simulink library "GPS_INS_Block"  (R2018b)
settings: Solver=VariableStepAuto  StartTime=0.0  StopTime=10.0  RelTol=1e-3
undefined symbols (not defined in the file): ac1dyn_alt0_ft, ac1dyn_lat0_rad, ac1dyn_lon0_rad, magnitude, uas_own_altQuant_ft, uas_own_dt_s, uas_own_phi_random_stddev_rad, uas_own_psi_random_stddev_rad, uas_own_seed1, uas_own_seed10, uas_own_seed2, uas_own_seed3, uas_own_seed4, uas_own_seed5, uas_own_seed6, uas_own_seed7, uas_own_seed8, uas_own_seed9, uas_own_theta_random_stddev_rad, uas_own_usePerfectAlt, uas_own_vx_bias_ftps, uas_own_vx_random_stddev_ftps, uas_own_vx_tau_s, uas_own_vy_bias_ftps, uas_own_vy_random_stddev_ftps, uas_own_vy_tau_s, uas_own_x_bias_ft, uas_own_x_random_stddev_ft, uas_own_x_tau_s, uas_own_y_bias_ft, uas_own_y_random_stddev_ft, uas_own_y_tau_s
libraries: simulink x4, TSAA_AltRate_Error x1, TSAA_Altitude_Error x1
settings Model: Creator=RA24876  LastModifiedBy=BI28030
settings SFSimCC: SimUseLocalCustomCode=off
settings RTWCC: RTWUseLocalCustomCode=off
settings CodeAppCC: StateflowObjectComments=on

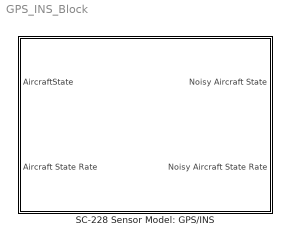
== system GPS_INS_Block ==
  SC-228 Sensor Model: GPS/INS : Subsystem  mask(Own State: GPS){dt_s=uas_own_dt_s, perfect=uas_own_usePerfectAlt, lat0_rad=ac1dyn_lat0_rad, lon0_rad=ac1dyn_lon0_rad, alt0_ft=ac1dyn_alt0_ft, vx_random_stddev_ftps=uas_own_vy_random_stddev_ftps, vx_bias_ftps=uas_own_vy_bias_ftps, vx_tau_s=uas_own_vy_tau_s, seed4=uas_own_seed4, vy_random_stddev_ftps=uas_own_vx_random_stddev_ftps, vy_bias_ftps=uas_own_vx_bias_ftps, vy_tau_s=uas_own_vx_tau_s, seed5=uas_own_seed5, psi_random_stddev_rad=uas_own_psi_random_stddev_rad, seed1=uas_own_seed1, phi_random_stddev_rad=uas_own_phi_random_stddev_rad, seed2=uas_own_seed2, theta_random_stddev_rad=uas_own_theta_random_stddev_rad, seed3=uas_own_seed3, seed6=uas_own_seed6, y_random_stddev_ft=uas_own_y_random_stddev_ft, y_bias_ft=uas_own_y_bias_ft, y_tau_s=uas_own_y_tau_s, seed7=uas_own_seed7, x_random_stddev_ft=uas_own_x_random_stddev_ft, x_bias_ft=uas_own_x_bias_ft, x_tau_s=uas_own_x_tau_s, seed8=uas_own_seed8, seed9=uas_own_seed9, seed10=uas_own_seed10, altQuant_ft=uas_own_altQuant_ft}
      mask prompts: dt_s "Timestep (s)"; perfect "Use Perfect Altimetry?"; lat0_rad "ENU Reference Latitude (rad)"; lon0_rad "ENU Reference Longitude (rad)"; alt0_ft "ENU Reference Altitude (ft)"; vx_random_stddev_ftps "Random Error Standard Deviation (ft/s)"; vx_bias_ftps "Bias Error (ft/s)"; vx_tau_s "Correlation Time (s)"; seed4 "Random Seed"; vy_random_stddev_ftps "Random Error Standard Deviation (ft/s)"; vy_bias_ftps "Bias Error (ft/s)"; vy_tau_s "Correlation Time (s)"; seed5 "Random Seed"; psi_random_stddev_rad "Random Error Standard Deviation (rad)"; seed1 "Random Seed"; phi_random_stddev_rad "Random Error Standard Deviation (rad)"; seed2 "Random Seed"; theta_random_stddev_rad "Random Error Standard Deviation (rad)"; seed3 "Random Seed"; seed6 "Random Seed"; y_random_stddev_ft "Random Error Standard Deviation (ft)"; y_bias_ft "Bias Error (ft)"; y_tau_s "Correlation Time (s)"; seed7 "Random Seed"; x_random_stddev_ft "Random Error Standard Deviation (ft)"; x_bias_ft "Bias Error (ft)"; x_tau_s "Correlation Time (s)"; seed8 "Random Seed"; seed9 "Lambda Random Seed"; seed10 "Random Seed"; altQuant_ft "Altitude Quantization"
      mask help: Ownship navigation error model with colored noise with state and state rate output.
      mask Help:
      | Additive noise model of ownship GPS navigation.  Independent noise is added to
      | each of latitude, longitude, and altitude and their rates as well as vertical acceleration,
      | heading, roll, and roll rate parameters. Noise is colored using weights determined
      | by time constant parameters.
      | 
      | Output takes the form of AircraftState and AircraftStateRate data buses.
      mask DialogControl ParameterTabVar0 Prompt: Tab
      mask DialogControl ParameterTabVar01234 Prompt: Velocity (N)
      mask DialogControl ParameterTabVar012345 Prompt: Velocity (E)
      mask DialogControl ParameterTabVar012345678 Prompt: Heading
      mask DialogControl ParameterTabVar0123456789 Prompt: Roll
      mask DialogControl ParameterTabVar012345678910 Prompt: Pitch
      mask DialogControl ParameterTabVar012345678911 Prompt: Vertical Rate
      mask DialogControl ParameterTabVar012345678912 Prompt: Position (N)
      mask DialogControl ParameterTabVar012345678913 Prompt: Position (E)
      mask DialogControl ParameterTabVar012345678914 Prompt: Position (h)

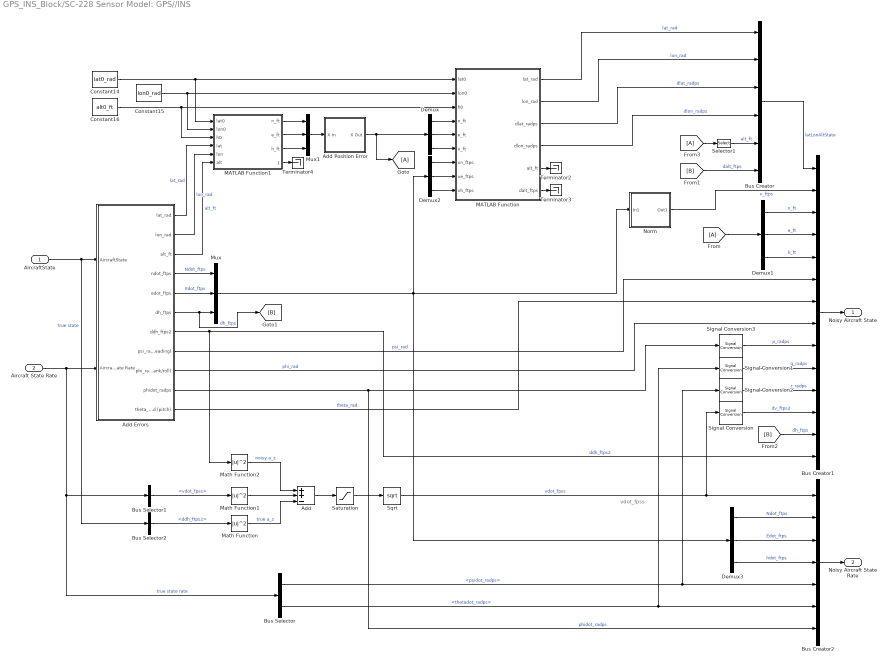
== system GPS_INS_Block/SC-228 Sensor Model: GPS//INS ==
  note: vdot_fpss
  AircraftState : Inport  OutDataTypeStr=Bus: AircraftState
  Aircraft State Rate : Inport  Port=2  OutDataTypeStr=Bus: AircraftStateRate
  Add : Sum  Inputs=++-
  Add Errors : Subsystem
  Add Position Error : Subsystem
  Bus Creator : BusCreator  Inputs=6  OutDataTypeStr=Bus: LatLonAltMeasurement
  Bus Creator1 : BusCreator  Inputs=14  OutDataTypeStr=Bus: AircraftState
  Bus Creator2 : BusCreator  Inputs=7  OutDataTypeStr=Bus: AircraftStateRate
  Bus Selector : BusSelector  OutputSignals=psidot_radps,thetadot_radps
  Bus Selector1 : BusSelector  OutputSignals=vdot_fpss
  Bus Selector2 : BusSelector  OutputSignals=ddh_ftps2
  Constant14 : Constant  Value=lat0_rad  OutDataTypeStr=double
  Constant15 : Constant  Value=lon0_rad  OutDataTypeStr=double
  Constant16 : Constant  Value=alt0_ft  OutDataTypeStr=double
  Demux{,1..3} (4 alike) : Demux  Outputs=3
  MATLAB Function : MATLAB Function  TreatAsAtomicUnit=on
  MATLAB Function1 : MATLAB Function  TreatAsAtomicUnit=on
  Math Function : Math  Operator=magnitude^2  SaturateOnIntegerOverflow=on
  Math Function1 : Math  Operator=magnitude^2  SaturateOnIntegerOverflow=on
  Math Function2 : Math  Operator=magnitude^2  SaturateOnIntegerOverflow=on
  Mux : Mux  Inputs=3
  Mux1 : Mux  Inputs=3
  Norm : Subsystem
  Saturation : Saturate  UpperLimit=Inf  LowerLimit=0
  Selector1 : Selector  InputPortWidth=3  IndexOptions=Index vector (dialog)  Indices=[3]  OutputSizes=1
  Signal Conversion{,1..3} (4 alike) : SignalConversion  OverrideOpt=off
  Sqrt : Sqrt  SaturateOnIntegerOverflow=on
  Terminator2 : Terminator
  Terminator3 : Terminator
  Terminator4 : Terminator
  Noisy Aircraft State : Outport  OutDataTypeStr=Bus: AircraftState
  Noisy Aircraft State Rate : Outport  Port=2  OutDataTypeStr=Bus: AircraftStateRate
  wires:
  Signal Conversion3/1 -> Bus Creator1/9  "p_radps"
  Signal Conversion2/1 -> Bus Creator1/11  "r_radps"
  Signal Conversion1/1 -> Bus Creator1/10  "q_radps"
  Add Errors/11(theta_rad (pitch)) -> Bus Creator1/7  "theta_rad"
  [B] -> Bus Creator1/13  "dh_ftps"
  [B] -> Bus Creator/6  "dalt_ftps"
  Demux3/3 -> Bus Creator2/4  "hdot_ftps"
  Demux3/2 -> Bus Creator2/3  "Edot_ftps"
  Demux3/1 -> Bus Creator2/2  "Ndot_ftps"
  Demux2/3 -> MATLAB Function/9(vh_ftps)
  Demux2/2 -> MATLAB Function/8(ve_ftps)
  Demux2/1 -> MATLAB Function/7(vn_ftps)
  Demux1/1 -> Bus Creator1/3  "n_ft"
  Demux1/2 -> Bus Creator1/4  "e_ft"
  Demux1/3 -> Bus Creator1/5  "h_ft"
  Mux1/1 -> Add Position Error/1(X In)
  Demux/3 -> MATLAB Function/6(u_ft)
  Demux/2 -> MATLAB Function/5(e_ft)
  Demux/1 -> MATLAB Function/4(n_ft)
  Signal Conversion/1 -> Bus Creator1/12  "dv_ftps2"
  Norm/1(Out1) -> Bus Creator1/2  "v_ftps"
  Mux/1 -> Demux3/1, Norm/1(In1), Demux2/1
  Sqrt/1 -> Signal Conversion/1, Bus Creator2/1  "vdot_fpss"
  Add/1 -> Saturation/1
  Math Function/1 -> Add/3  "true a_z"
  Math Function2/1 -> Add/1  "noisy a_z"
  Math Function1/1 -> Add/2
  Bus Selector2/1 -> Math Function/1  "<ddh_ftps2>"
  Bus Selector1/1 -> Math Function1/1  "<vdot_fpss>"
  Constant14/1 -> MATLAB Function1/1(lat0), MATLAB Function/1(lat0)
  Constant15/1 -> MATLAB Function1/2(lon0), MATLAB Function/2(lon0)
  Constant16/1 -> MATLAB Function1/3(h0), MATLAB Function/3(h0)
  MATLAB Function1/3(h_ft) -> Mux1/3
  MATLAB Function1/2(e_ft) -> Mux1/2
  MATLAB Function1/1(n_ft) -> Mux1/1
  MATLAB Function1/4(J) -> Terminator4/1
  MATLAB Function/4(dlon_radps) -> Bus Creator/4  "dlon_radps"
  MATLAB Function/3(dlat_radps) -> Bus Creator/3  "dlat_radps"
  Bus Selector/2 -> Bus Creator2/6, Signal Conversion1/1  "<thetadot_radps>"
  Bus Selector/1 -> Signal Conversion2/1, Bus Creator2/5  "<psidot_radps>"
  Add Errors/5(edot_ftps) -> Mux/2  "Edot_ftps"
  Add Errors/4(ndot_ftps) -> Mux/1  "Ndot_ftps"
  Bus Creator2/1 -> Noisy Aircraft State Rate/1
  Bus Creator1/1 -> Noisy Aircraft State/1
  Bus Creator/1 -> Bus Creator1/1  "latLonAltState"
  MATLAB Function/6(dalt_ftps) -> Terminator3/1
  MATLAB Function/5(alt_ft) -> Terminator2/1
  Add Errors/6(dh_ftps) -> Mux/3, [B]  "dh_ftps"
  Add Errors/3(alt_ft) -> MATLAB Function1/6(alt)  "alt_ft"
  Add Errors/2(lon_rad) -> MATLAB Function1/5(lon)  "lon_rad"
  Add Errors/1(lat_rad) -> MATLAB Function1/4(lat)  "lat_rad"
  Add Errors/10(phidot_radps) -> Bus Creator2/7, Signal Conversion3/1  "phidot_radps"
  Add Errors/9(phi_rad (bank/roll)) -> Bus Creator1/8  "phi_rad"
  Add Errors/8(psi_rad (heading)) -> Bus Creator1/6  "psi_rad"
  Add Errors/7(ddh_ftps2) -> Bus Creator1/14, Math Function2/1  "ddh_ftps2"
  Aircraft State Rate/1 -> Add Errors/2(Aircraft State Rate), Bus Selector1/1, Bus Selector/1  "true state rate"
  AircraftState/1 -> Add Errors/1(AircraftState), Bus Selector2/1  "true state"
  Saturation/1 -> Sqrt/1
  Add Position Error/1(X Out) -> Demux/1, [A]
  [A] -> Selector1/1
  Selector1/1 -> Bus Creator/5  "alt_ft"
  [A] -> Demux1/1
  MATLAB Function/1(lat_rad) -> Bus Creator/1  "lat_rad"
  MATLAB Function/2(lon_rad) -> Bus Creator/2  "lon_rad"

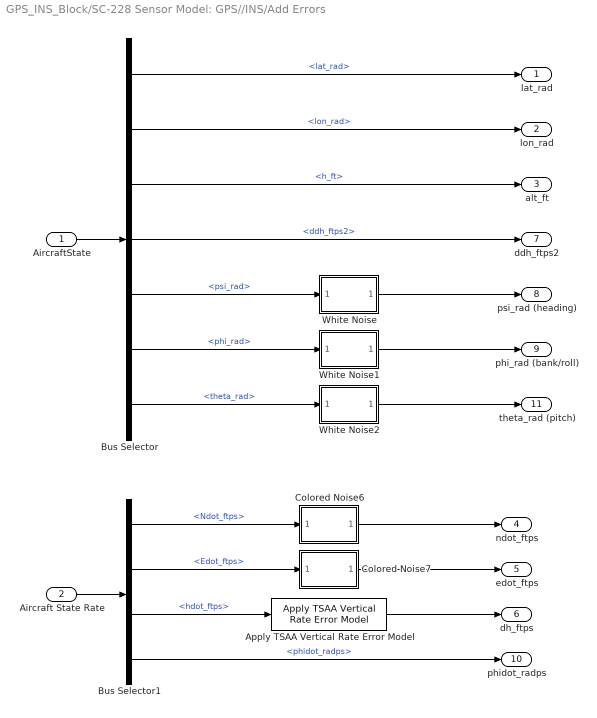
== system GPS_INS_Block/SC-228 Sensor Model: GPS//INS/Add Errors ==
  AircraftState : Inport  OutDataTypeStr=Bus: AircraftState
  Aircraft State Rate : Inport  Port=2  OutDataTypeStr=Bus: AircraftStateRate
  Apply TSAA Vertical Rate Error Model : TSAA_AltRate_Error/Apply TSAA Vertical Rate Error Model  perfect=perfect  seed=seed6  dt_s=dt_s
  Bus Selector : BusSelector  OutputSignals=latLonAltState.lat_rad,latLonAltState.lon_rad,h_ft,ddh_ftps2,psi_rad,phi_rad,theta_rad
  Bus Selector1 : BusSelector  OutputSignals=Ndot_ftps,Edot_ftps,hdot_ftps,phidot_radps
  Colored Noise6 : Subsystem  mask(Colored Noise){sig=vy_random_stddev_ftps, bias=vy_bias_ftps, tau=vy_tau_s, dt=dt_s, seed=seed4}
      mask prompts: sig "Random error standard deviation"; bias "Bias error"; tau "Correlation time"; dt "Track update time"; seed "Random Seed"
      mask help: Generates a noisy state variable estimate using the ABSAA colored noise model. Set correlation time to zero for white noise.
      mask Help:
      | Generates a noisy state variable estimate using the AF Common ABSAA error
      | model.  Time correlation of the error is defined by an exponential decay
      | of K = exp(-tau/dt), where tau is the correlation time and dt is the time
      | between track updates.  The track error at time t is then:
      | 
      |     err(t) = K*err(t-1) + N(0,(1-K^2)*sig^2) + bias
      | 
      | where N(x,y) is a Gaussian noise process with mean x and variance y and
      | with random number generator seeded with the integer 'seed'.
      | 
      | The random noise process must be initialized with an error drawn from
      | N(0,sig^2).
      | 
      | The noise model can be used to produce white noise by setting tau to zero.
  Colored Noise7 : Subsystem  mask(Colored Noise){sig=vx_random_stddev_ftps, bias=vx_bias_ftps, tau=vx_tau_s, dt=dt_s, seed=seed5}
      mask prompts: sig "Random error standard deviation"; bias "Bias error"; tau "Correlation time"; dt "Track update time"; seed "Random Seed"
      mask help: Generates a noisy state variable estimate using the ABSAA colored noise model. Set correlation time to zero for white noise.
      mask Help:
      | Generates a noisy state variable estimate using the AF Common ABSAA error
      | model.  Time correlation of the error is defined by an exponential decay
      | of K = exp(-tau/dt), where tau is the correlation time and dt is the time
      | between track updates.  The track error at time t is then:
      | 
      |     err(t) = K*err(t-1) + N(0,(1-K^2)*sig^2) + bias
      | 
      | where N(x,y) is a Gaussian noise process with mean x and variance y and
      | with random number generator seeded with the integer 'seed'.
      | 
      | The random noise process must be initialized with an error drawn from
      | N(0,sig^2).
      | 
      | The noise model can be used to produce white noise by setting tau to zero.
  White Noise : Subsystem  mask(Colored Noise){sig=psi_random_stddev_rad, seed=seed1}
      mask prompts: sig "Random error standard deviation"; seed "Random Seed"
      mask help: Generates a noisy state variable estimate using the ABSAA colored noise model. Set correlation time to zero for white noise.
      mask Help:
      | Generates a noisy state variable estimate using the AF Common ABSAA error
      | model.  Time correlation of the error is defined by an exponential decay
      | of K = exp(-tau/dt), where tau is the correlation time and dt is the time
      | between track updates.  The track error at time t is then:
      | 
      |     err(t) = K*err(t-1) + N(0,(1-K^2)*sig^2) + bias
      | 
      | where N(x,y) is a Gaussian noise process with mean x and variance y and
      | with random number generator seeded with the integer 'seed'.
      | 
      | The random noise process must be initialized with an error drawn from
      | N(0,sig^2).
      | 
      | The noise model can be used to produce white noise by setting tau to zero.
  White Noise1 : Subsystem  mask(Colored Noise){sig=phi_random_stddev_rad, seed=seed2}
      mask prompts: sig "Random error standard deviation"; seed "Random Seed"
      mask help: Generates a noisy state variable estimate using the ABSAA colored noise model. Set correlation time to zero for white noise.
      mask Help:
      | Generates a noisy state variable estimate using the AF Common ABSAA error
      | model.  Time correlation of the error is defined by an exponential decay
      | of K = exp(-tau/dt), where tau is the correlation time and dt is the time
      | between track updates.  The track error at time t is then:
      | 
      |     err(t) = K*err(t-1) + N(0,(1-K^2)*sig^2) + bias
      | 
      | where N(x,y) is a Gaussian noise process with mean x and variance y and
      | with random number generator seeded with the integer 'seed'.
      | 
      | The random noise process must be initialized with an error drawn from
      | N(0,sig^2).
      | 
      | The noise model can be used to produce white noise by setting tau to zero.
  White Noise2 : Subsystem  mask(Colored Noise){sig=theta_random_stddev_rad, seed=seed3}
      mask prompts: sig "Random error standard deviation"; seed "Random Seed"
      mask help: Generates a noisy state variable estimate using the ABSAA colored noise model. Set correlation time to zero for white noise.
      mask Help:
      | Generates a noisy state variable estimate using the AF Common ABSAA error
      | model.  Time correlation of the error is defined by an exponential decay
      | of K = exp(-tau/dt), where tau is the correlation time and dt is the time
      | between track updates.  The track error at time t is then:
      | 
      |     err(t) = K*err(t-1) + N(0,(1-K^2)*sig^2) + bias
      | 
      | where N(x,y) is a Gaussian noise process with mean x and variance y and
      | with random number generator seeded with the integer 'seed'.
      | 
      | The random noise process must be initialized with an error drawn from
      | N(0,sig^2).
      | 
      | The noise model can be used to produce white noise by setting tau to zero.
  lat_rad : Outport
  lon_rad : Outport  Port=2
  alt_ft : Outport  Port=3
  ndot_ftps : Outport  Port=4
  edot_ftps : Outport  Port=5
  dh_ftps : Outport  Port=6
  ddh_ftps2 : Outport  Port=7
  psi_rad (heading) : Outport  Port=8
  phi_rad (bank/roll) : Outport  Port=9
  phidot_radps : Outport  Port=10
  theta_rad (pitch) : Outport  Port=11
  wires:
  Bus Selector1/1 -> Colored Noise6/1(truth)  "<Ndot_ftps>"
  Bus Selector1/2 -> Colored Noise7/1(truth)  "<Edot_ftps>"
  Bus Selector1/3 -> Apply TSAA Vertical Rate Error Model/1  "<hdot_ftps>"
  Bus Selector1/4 -> phidot_radps/1  "<phidot_radps>"
  Aircraft State Rate/1 -> Bus Selector1/1
  Colored Noise6/1(noisy) -> ndot_ftps/1
  White Noise/1(noisy) -> psi_rad (heading)/1
  Bus Selector/4 -> ddh_ftps2/1  "<ddh_ftps2>"
  Bus Selector/1 -> lat_rad/1  "<lat_rad>"
  Colored Noise7/1(noisy) -> edot_ftps/1
  AircraftState/1 -> Bus Selector/1
  Bus Selector/6 -> White Noise1/1(truth)  "<phi_rad>"
  Bus Selector/2 -> lon_rad/1  "<lon_rad>"
  Bus Selector/5 -> White Noise/1(truth)  "<psi_rad>"
  White Noise1/1(noisy) -> phi_rad (bank/roll)/1
  Bus Selector/3 -> alt_ft/1  "<h_ft>"
  Apply TSAA Vertical Rate Error Model/1 -> dh_ftps/1
  Bus Selector/7 -> White Noise2/1(truth)  "<theta_rad>"
  White Noise2/1(noisy) -> theta_rad (pitch)/1

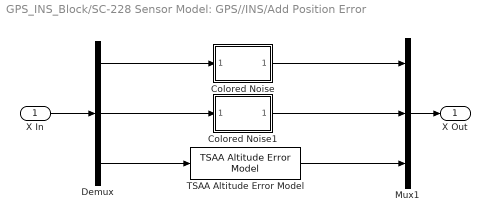
== system GPS_INS_Block/SC-228 Sensor Model: GPS//INS/Add Position Error ==
  X In : Inport
  Colored Noise : Subsystem  mask(Colored Noise){sig=y_random_stddev_ft, bias=y_bias_ft, tau=y_tau_s, dt=dt_s, seed=seed7}
      mask prompts: sig "Random error standard deviation"; bias "Bias error"; tau "Correlation time"; dt "Track update time"; seed "Random Seed"
      mask help: Generates a noisy state variable estimate using the ABSAA colored noise model. Set correlation time to zero for white noise.
      mask Help:
      | Generates a noisy state variable estimate using the AF Common ABSAA error
      | model.  Time correlation of the error is defined by an exponential decay
      | of K = exp(-tau/dt), where tau is the correlation time and dt is the time
      | between track updates.  The track error at time t is then:
      | 
      |     err(t) = K*err(t-1) + N(0,(1-K^2)*sig^2) + bias
      | 
      | where N(x,y) is a Gaussian noise process with mean x and variance y and
      | with random number generator seeded with the integer 'seed'.
      | 
      | The random noise process must be initialized with an error drawn from
      | N(0,sig^2).
      | 
      | The noise model can be used to produce white noise by setting tau to zero.
  Colored Noise1 : Subsystem  mask(Colored Noise){sig=x_random_stddev_ft, bias=x_bias_ft, tau=x_tau_s, dt=dt_s, seed=seed8}
      mask prompts: sig "Random error standard deviation"; bias "Bias error"; tau "Correlation time"; dt "Track update time"; seed "Random Seed"
      mask help: Generates a noisy state variable estimate using the ABSAA colored noise model. Set correlation time to zero for white noise.
      mask Help:
      | Generates a noisy state variable estimate using the AF Common ABSAA error
      | model.  Time correlation of the error is defined by an exponential decay
      | of K = exp(-tau/dt), where tau is the correlation time and dt is the time
      | between track updates.  The track error at time t is then:
      | 
      |     err(t) = K*err(t-1) + N(0,(1-K^2)*sig^2) + bias
      | 
      | where N(x,y) is a Gaussian noise process with mean x and variance y and
      | with random number generator seeded with the integer 'seed'.
      | 
      | The random noise process must be initialized with an error drawn from
      | N(0,sig^2).
      | 
      | The noise model can be used to produce white noise by setting tau to zero.
  Demux : Demux  Outputs=3
  Mux1 : Mux  Inputs=3
  TSAA Altitude Error Model : TSAA_Altitude_Error/TSAA Altitude Error Model  ac_id=1  perfect=perfect  lambdaSeed=seed9  randomSeed=seed10  altQuant_ft=altQuant_ft  dt_s=dt_s
  X Out : Outport
  wires:
  Mux1/1 -> X Out/1
  X In/1 -> Demux/1
  Demux/3 -> TSAA Altitude Error Model/1
  TSAA Altitude Error Model/1 -> Mux1/3
  Demux/1 -> Colored Noise/1(truth)
  Colored Noise/1(noisy) -> Mux1/1
  Demux/2 -> Colored Noise1/1(truth)
  Colored Noise1/1(noisy) -> Mux1/2

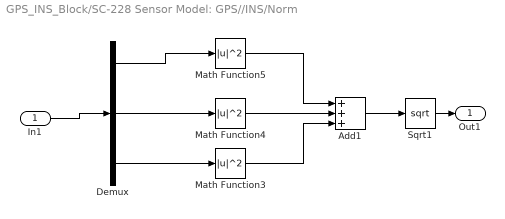
== system GPS_INS_Block/SC-228 Sensor Model: GPS//INS/Norm ==
  In1 : Inport
  Add1 : Sum  Inputs=+++
  Demux : Demux  Outputs=3
  Math Function3 : Math  Operator=magnitude^2  SaturateOnIntegerOverflow=on
  Math Function4 : Math  Operator=magnitude^2  SaturateOnIntegerOverflow=on
  Math Function5 : Math  Operator=magnitude^2  SaturateOnIntegerOverflow=on
  Sqrt1 : Sqrt  SaturateOnIntegerOverflow=on
  Out1 : Outport
  wires:
  In1/1 -> Demux/1
  Demux/2 -> Math Function4/1
  Math Function3/1 -> Add1/3
  Math Function4/1 -> Add1/2
  Math Function5/1 -> Add1/1
  Demux/3 -> Math Function3/1
  Sqrt1/1 -> Out1/1
  Demux/1 -> Math Function5/1
  Add1/1 -> Sqrt1/1

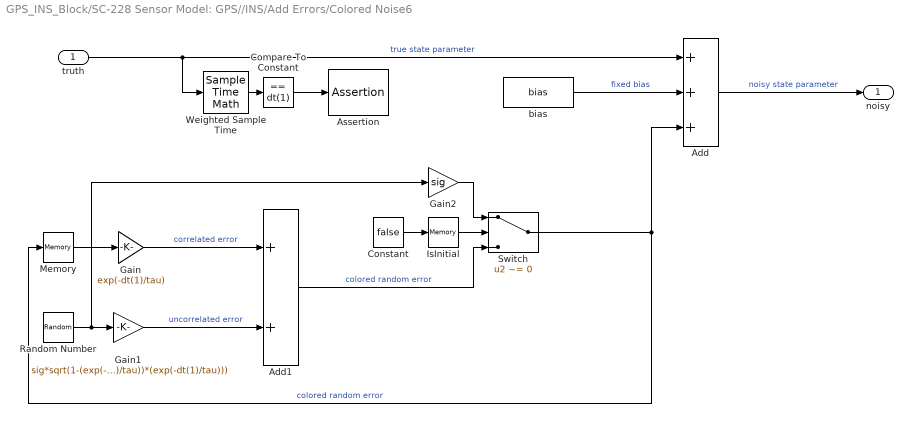
== system GPS_INS_Block/SC-228 Sensor Model: GPS//INS/Add Errors/Colored Noise6 ==
  truth : Inport
  Add : Sum  Inputs=+++  SampleTime=dt_s
  Add1 : Sum  SampleTime=dt
  Assertion : Assertion
  Compare To Constant : simulink/Logic and Bit Operations/Compare To Constant  relop===  const=dt(1)  OutDataTypeStr=boolean
  Constant : Constant  Value=false
  Gain : Gain  Gain=exp(-dt(1)/tau)  SampleTime=dt
  Gain1 : Gain  Gain=sig*sqrt(1-(exp(-dt(1)/tau))*(exp(-dt(1)/tau)))
  Gain2 : Gain  Gain=sig
  IsInitial : Memory  InitialCondition=true  InheritSampleTime=on
  Memory : Memory  InheritSampleTime=on
  Random Number : RandomNumber  Seed=seed  SampleTime=dt_s
  Switch : Switch  Criteria=u2 ~= 0  SampleTime=dt
  Weighted Sample Time : SampleTimeMath  TsampMathOp=Ts Only
  bias : Constant  Value=bias
  noisy : Outport
  wires:
  Compare To Constant/1 -> Assertion/1
  Weighted Sample Time/1 -> Compare To Constant/1
  Gain2/1 -> Switch/1
  Add1/1 -> Switch/3  "colored random error"
  IsInitial/1 -> Switch/2
  Constant/1 -> IsInitial/1
  Memory/1 -> Gain/1
  truth/1 -> Add/1, Weighted Sample Time/1  "true state parameter"
  Add/1 -> noisy/1  "noisy state parameter"
  Gain/1 -> Add1/1  "correlated error"
  Random Number/1 -> Gain1/1, Gain2/1
  bias/1 -> Add/2  "fixed bias"
  Switch/1 -> Add/3, Memory/1  "colored random error"
  Gain1/1 -> Add1/2  "uncorrelated error"

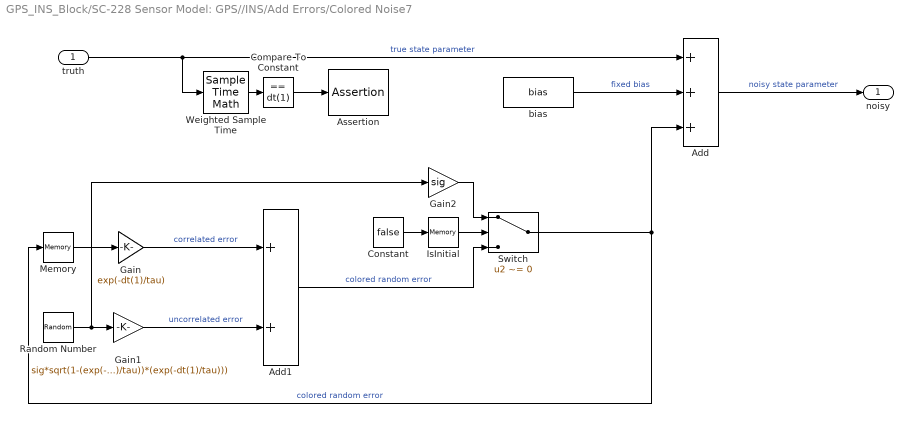
== system GPS_INS_Block/SC-228 Sensor Model: GPS//INS/Add Errors/Colored Noise7 ==
  truth : Inport
  Add : Sum  Inputs=+++  SampleTime=dt_s
  Add1 : Sum  SampleTime=dt
  Assertion : Assertion
  Compare To Constant : simulink/Logic and Bit Operations/Compare To Constant  relop===  const=dt(1)  OutDataTypeStr=boolean
  Constant : Constant  Value=false
  Gain : Gain  Gain=exp(-dt(1)/tau)  SampleTime=dt
  Gain1 : Gain  Gain=sig*sqrt(1-(exp(-dt(1)/tau))*(exp(-dt(1)/tau)))
  Gain2 : Gain  Gain=sig
  IsInitial : Memory  InitialCondition=true  InheritSampleTime=on
  Memory : Memory  InheritSampleTime=on
  Random Number : RandomNumber  Seed=seed  SampleTime=dt_s
  Switch : Switch  Criteria=u2 ~= 0  SampleTime=dt
  Weighted Sample Time : SampleTimeMath  TsampMathOp=Ts Only
  bias : Constant  Value=bias
  noisy : Outport
  wires:
  Compare To Constant/1 -> Assertion/1
  Weighted Sample Time/1 -> Compare To Constant/1
  Gain2/1 -> Switch/1
  Add1/1 -> Switch/3  "colored random error"
  IsInitial/1 -> Switch/2
  Constant/1 -> IsInitial/1
  Memory/1 -> Gain/1
  truth/1 -> Add/1, Weighted Sample Time/1  "true state parameter"
  Add/1 -> noisy/1  "noisy state parameter"
  Gain/1 -> Add1/1  "correlated error"
  Random Number/1 -> Gain1/1, Gain2/1
  bias/1 -> Add/2  "fixed bias"
  Switch/1 -> Add/3, Memory/1  "colored random error"
  Gain1/1 -> Add1/2  "uncorrelated error"

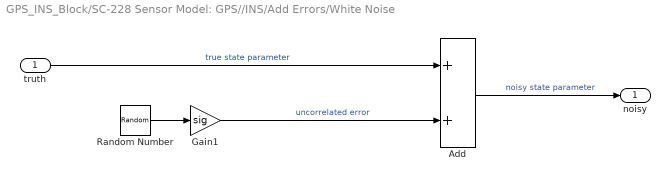
== system GPS_INS_Block/SC-228 Sensor Model: GPS//INS/Add Errors/White Noise ==
  truth : Inport
  Add : Sum  SampleTime=dt_s
  Gain1 : Gain  Gain=sig
  Random Number : RandomNumber  Seed=seed  SampleTime=dt_s
  noisy : Outport
  wires:
  truth/1 -> Add/1  "true state parameter"
  Add/1 -> noisy/1  "noisy state parameter"
  Random Number/1 -> Gain1/1
  Gain1/1 -> Add/2  "uncorrelated error"

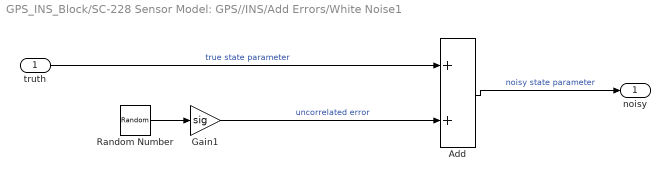
== system GPS_INS_Block/SC-228 Sensor Model: GPS//INS/Add Errors/White Noise1 ==
  truth : Inport
  Add : Sum  SampleTime=dt_s
  Gain1 : Gain  Gain=sig
  Random Number : RandomNumber  Seed=seed  SampleTime=dt_s
  noisy : Outport
  wires:
  Gain1/1 -> Add/2  "uncorrelated error"
  Random Number/1 -> Gain1/1
  Add/1 -> noisy/1  "noisy state parameter"
  truth/1 -> Add/1  "true state parameter"

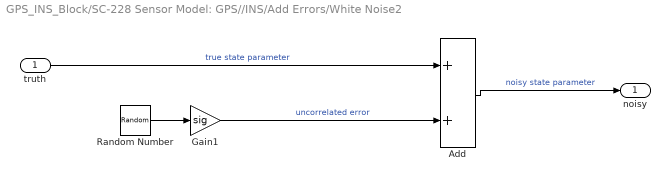
== system GPS_INS_Block/SC-228 Sensor Model: GPS//INS/Add Errors/White Noise2 ==
  truth : Inport
  Add : Sum  SampleTime=dt_s
  Gain1 : Gain  Gain=sig
  Random Number : RandomNumber  Seed=seed  SampleTime=dt_s
  noisy : Outport
  wires:
  truth/1 -> Add/1  "true state parameter"
  Add/1 -> noisy/1  "noisy state parameter"
  Random Number/1 -> Gain1/1
  Gain1/1 -> Add/2  "uncorrelated error"

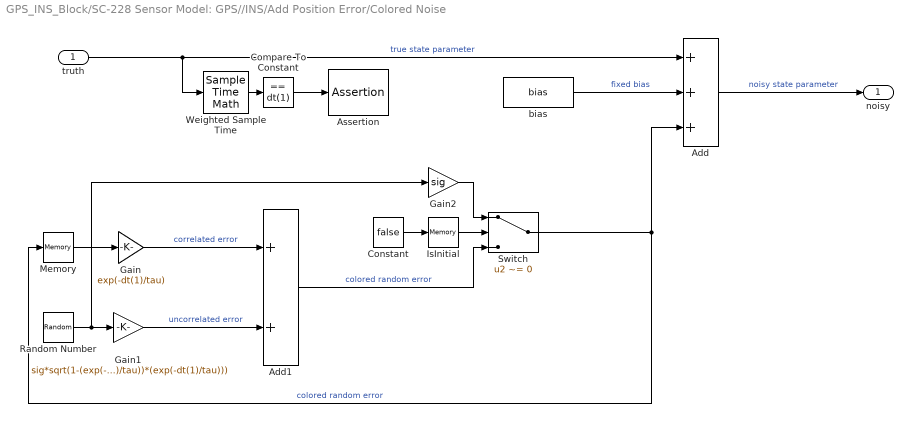
== system GPS_INS_Block/SC-228 Sensor Model: GPS//INS/Add Position Error/Colored Noise ==
  truth : Inport
  Add : Sum  Inputs=+++  SampleTime=dt
  Add1 : Sum  SampleTime=dt
  Assertion : Assertion
  Compare To Constant : simulink/Logic and Bit Operations/Compare To Constant  relop===  const=dt(1)  OutDataTypeStr=boolean
  Constant : Constant  Value=false
  Gain : Gain  Gain=exp(-dt(1)/tau)  SampleTime=dt
  Gain1 : Gain  Gain=sig*sqrt(1-(exp(-dt(1)/tau))*(exp(-dt(1)/tau)))
  Gain2 : Gain  Gain=sig
  IsInitial : Memory  InitialCondition=true  InheritSampleTime=on
  Memory : Memory  InheritSampleTime=on
  Random Number : RandomNumber  Seed=seed  SampleTime=dt_s
  Switch : Switch  Criteria=u2 ~= 0  SampleTime=dt
  Weighted Sample Time : SampleTimeMath  TsampMathOp=Ts Only
  bias : Constant  Value=bias
  noisy : Outport
  wires:
  Compare To Constant/1 -> Assertion/1
  Weighted Sample Time/1 -> Compare To Constant/1
  Gain2/1 -> Switch/1
  Add1/1 -> Switch/3  "colored random error"
  IsInitial/1 -> Switch/2
  Constant/1 -> IsInitial/1
  Memory/1 -> Gain/1
  truth/1 -> Add/1, Weighted Sample Time/1  "true state parameter"
  Add/1 -> noisy/1  "noisy state parameter"
  Gain/1 -> Add1/1  "correlated error"
  Random Number/1 -> Gain1/1, Gain2/1
  bias/1 -> Add/2  "fixed bias"
  Switch/1 -> Add/3, Memory/1  "colored random error"
  Gain1/1 -> Add1/2  "uncorrelated error"

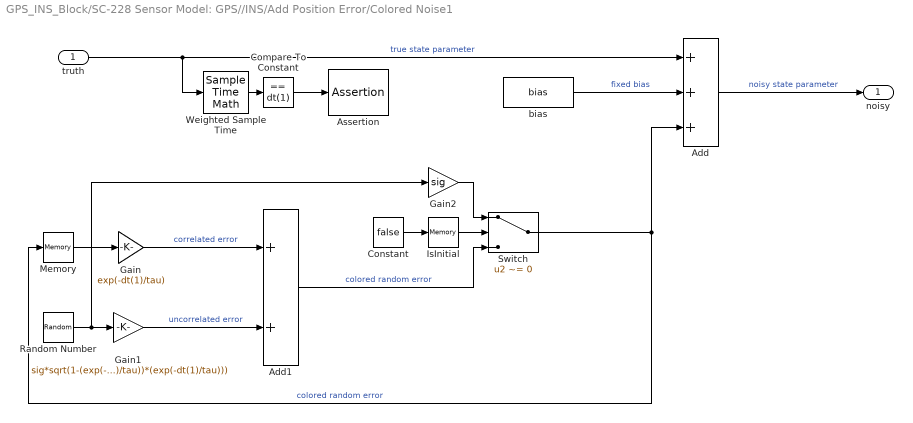
== system GPS_INS_Block/SC-228 Sensor Model: GPS//INS/Add Position Error/Colored Noise1 ==
  truth : Inport
  Add : Sum  Inputs=+++  SampleTime=dt
  Add1 : Sum  SampleTime=dt
  Assertion : Assertion
  Compare To Constant : simulink/Logic and Bit Operations/Compare To Constant  relop===  const=dt(1)  OutDataTypeStr=boolean
  Constant : Constant  Value=false
  Gain : Gain  Gain=exp(-dt(1)/tau)  SampleTime=dt
  Gain1 : Gain  Gain=sig*sqrt(1-(exp(-dt(1)/tau))*(exp(-dt(1)/tau)))
  Gain2 : Gain  Gain=sig
  IsInitial : Memory  InitialCondition=true  InheritSampleTime=on
  Memory : Memory  InheritSampleTime=on
  Random Number : RandomNumber  Seed=seed  SampleTime=dt_s
  Switch : Switch  Criteria=u2 ~= 0  SampleTime=dt
  Weighted Sample Time : SampleTimeMath  TsampMathOp=Ts Only
  bias : Constant  Value=bias
  noisy : Outport
  wires:
  Gain1/1 -> Add1/2  "uncorrelated error"
  Switch/1 -> Memory/1, Add/3  "colored random error"
  bias/1 -> Add/2  "fixed bias"
  Random Number/1 -> Gain2/1, Gain1/1
  Gain/1 -> Add1/1  "correlated error"
  Add/1 -> noisy/1  "noisy state parameter"
  truth/1 -> Weighted Sample Time/1, Add/1  "true state parameter"
  Memory/1 -> Gain/1
  Constant/1 -> IsInitial/1
  IsInitial/1 -> Switch/2
  Add1/1 -> Switch/3  "colored random error"
  Gain2/1 -> Switch/1
  Weighted Sample Time/1 -> Compare To Constant/1
  Compare To Constant/1 -> Assertion/1

== matlab function GPS_INS_Block/SC-228 Sensor Model: GPS//INS/MATLAB Function ==
  data: lat0 input double; lon0 input double; h0 input double; n_ft input double; e_ft input double size=1; u_ft input double; vn_ftps input double; ve_ftps input double; vh_ftps input double; lat_rad output double; lon_rad output double; dlat_radps output double; dlon_radps output double; alt_ft output double; dalt_ftps output double
function [lat_rad,lon_rad,dlat_radps,dlon_radps,alt_ft,dalt_ftps] = convertToLLA(lat0,lon0,h0,n_ft,e_ft,u_ft,vn_ftps,ve_ftps,vh_ftps)
%#codegen

% WGS-84 ellipsoid constants
a = 2.09256*10^7;          %Semi-major axis (ft)
f = 1.0/298.257223563;  %Flattening
ecc_sq = f*(2.0-f);        %Eccentricity^2


% Ellipsoidal "radius"
er = a./sqrt(1-ecc_sq.*sin(lat0).^2);


% ECEF coordinates
x0 = (er + h0)*cos(lat0)*cos(lon0);
y0 = (er + h0)*cos(lat0)*sin(lon0);
z0 = (er.*(1-ecc_sq) + h0)*sin(lat0);


%% Rotation Matrix
posECEF0 = [x0;y0;z0];
% Compute the local Up unit vector
vHatU = posECEF0;
vHatU(3) = vHatU(3) ./ ((1-f)^2);
vHatU = vHatU ./ norm(vHatU);

% Compute the projection onto the local Up vector
pU = vHatU * vHatU';

% Compute the projection onto the local Tangent plane
pT = eye(size(pU)) - pU;

% Compute the local North unit vector
vHatZ = [0;0;1];
vHatN = pT * vHatZ;
vHatN = vHatN ./ norm(vHatN);

% Compute the local East unit vector
vHatE = cross(vHatN,vHatU);

% Compute ENU rotation matrix
rotMatENU = zeros(3,3);
rotMatENU(:,1) = vHatE;
rotMatENU(:,2) = vHatN;
rotMatENU(:,3) = vHatU;

tPosECEF = rotMatENU*[e_ft;n_ft;u_ft] + [x0;y0;z0];


%% ECEF to LLA
% WGS-84 derived parameters
b = (1-f).*a;                       %Semi-minor axis (meters)
ecc1_sq = (a.^2 - b.^2)./(a.^2);    %First eccentricity squared
ecc2_sq = (a.^2 - b.^2)./(b.^2);    %Second eccentricity squared


% Length of position vector in equatorial plane
rho = sqrt(tPosECEF(1).^2 + tPosECEF(2).^2);

% Auxillary angle
theta = atan( (tPosECEF(3).*a)./(rho.*b) );

lon_rad = atan2(tPosECEF(2),tPosECEF(1));
lat_rad = atan( (tPosECEF(3) + ecc2_sq.*b.*(sin(theta)).^3)./(rho - ecc1_sq.*a.*(cos(theta)).^3) );

ewRadCurv = a./sqrt(1-ecc1_sq.*sin(lat_rad).^2);

alt_ft = (rho./cos(lat_rad)) - ewRadCurv;


%% Velocities - Project 1 sec into future and use to estimate
dalt_ftps = vh_ftps; % Assume about the same


tPosECEF_1sec = rotMatENU*[e_ft+ve_ftps;...
                           n_ft+vn_ftps;...
                           u_ft] + ...
                           [x0;y0;z0];

% Length of position vector in equatorial plane
rho = sqrt(tPosECEF_1sec(1).^2 + tPosECEF_1sec(2).^2);

% Auxillary angle
theta = atan( (tPosECEF_1sec(3).*a)./(rho.*b) );

lon_rad_1sec = atan2(tPosECEF_1sec(2),tPosECEF_1sec(1));
lat_rad_1sec = atan( (tPosECEF_1sec(3) + ecc2_sq.*b.*(sin(theta)).^3)./(rho - ecc1_sq.*a.*(cos(theta)).^3) );

dlat_radps = lat_rad_1sec - lat_rad;
dlon_radps = lon_rad_1sec - lon_rad;
end

== matlab function GPS_INS_Block/SC-228 Sensor Model: GPS//INS/MATLAB Function1 ==
  data: lat0 input; lon0 input; h0 input; lat input; n_ft output; lon input; alt input; e_ft output; h_ft output; J output
function [n_ft, e_ft, h_ft, J] = convertToNED(lat0, lon0, h0, lat, lon, alt)
%#codegen

% WGS-84 ellipsoid constants
a = 2.09256*10^7;          %Semi-major axis (ft)
f = 1.0/298.257223563;  %Flattening
ecc_sq = f*(2.0-f);        %Eccentricity^2

% Ellipsoidal "radius"
er = a./sqrt(1-ecc_sq.*sin(lat0).^2);

% ECEF coordinates of reference
x0 = (er + h0)*cos(lat0)*cos(lon0);
y0 = (er + h0)*cos(lat0)*sin(lon0);
z0 = (er.*(1-ecc_sq) + h0)*sin(lat0);

% Ellipsoidal "radius"
er = a./sqrt(1-ecc_sq.*sin(lat).^2);

% ECEF coordinates
x1 = (er + alt)*cos(lat)*cos(lon);
y1 = (er + alt)*cos(lat)*sin(lon);
z1 = (er.*(1-ecc_sq) + alt)*sin(lat);
xRelECEF = [x1-x0; y1-y0; z1-z0];

% convert to NED
dwn = -[x0; y0; z0];
dwn = dwn./norm(dwn);
east = cross(dwn,[0;0;1]);
east = east./norm(east);
north = cross(east,dwn);
north = north./norm(north);

T = [north'; east'; dwn'];

xRelENU = T*xRelECEF;

n_ft = xRelENU(1);
e_ft = xRelENU(2);
h_ft = alt;

% Jacobian (for conversion to ECEF, then use T to transform to NED)
der_dlat = a*ecc_sq*sin(lat)*cos(lat)/(1-ecc_sq*sin(lat)^2)^(3/2);

J = zeros(3);
J(1,1) = der_dlat*cos(lat)*cos(lon) - (er + alt)*sin(lat)*cos(lon);
J(1,2) = -(er + alt)*cos(lat)*sin(lon);
J(1,3) = cos(lat)*cos(lon);
J(2,1) = der_dlat*cos(lat)*sin(lon) - (er + alt)*sin(lat)*sin(lon);
J(2,2) = (er + alt)*cos(lat)*cos(lon);
J(2,3) = cos(lat)*sin(lon);
J(3,1) = (1-ecc_sq)*der_dlat*sin(lat) + ((1-ecc_sq)*er + alt)*cos(lat);
J(3,2) = 0;
J(3,3) = sin(lat);

J = T*J;
